simulink model "test"  (R2023b)
settings: Solver=VariableStepAuto  StartTime=0.0  StopTime=10.0  RelTol=1e-3
values from neighbouring files (symbols this model uses):
  f = 50    [model_script.m]    (also in setup_environment.m; test_setup.m)
  l = x./(2*pi*f)    [model_script.m]    (also in setup_environment.m; test_calc.m = 4e-07; test_setup.m = 4e-07)
  l1 = 3    [model_script.m]    (also in setup_environment.m; test_setup.m)
  l2 = 3.5    [model_script.m]    (also in setup_environment.m; test_setup.m = 5)
  l3 = 1.8    [model_script.m]    (also in setup_environment.m; test_setup.m = 8)
  l4 = 15    [test_setup.m]
  L_S = 16E-3    (= 0.016)    [model_script.m]    (also in setup_environment.m; test_setup.m = 0.01658)
  m_actual = 0.2    [model_script.m]    (also in run_sim.m = m_value(jjj); setup_environment.m; test_setup.m = 0.4)
  r = 0.4013    [model_script.m]    (also in setup_environment.m; test_calc.m = 0.4; test_setup.m = 0.4)
  R_S = 0.8913    [model_script.m]    (also in setup_environment.m; test_setup.m = 0.8929)
  trigger = [0 0 0 0]    [test_setup.m]
  V_S = 11000    [model_script.m]    (also in setup_environment.m; test_setup.m)
libraries: spsThreePhaseSeriesRLCBranchLib x8, spsThreePhaseSeriesRLCLoadLib x4, spsThreePhaseFaultLib x4, spsThreePhaseVIMeasurementLib x1, spsThreePhaseSourceLib x1, spsVoltageMeasurementLib x1, sps_lib x1
settings Model: Creator=CoolBose  LastModifiedBy=CoolBose

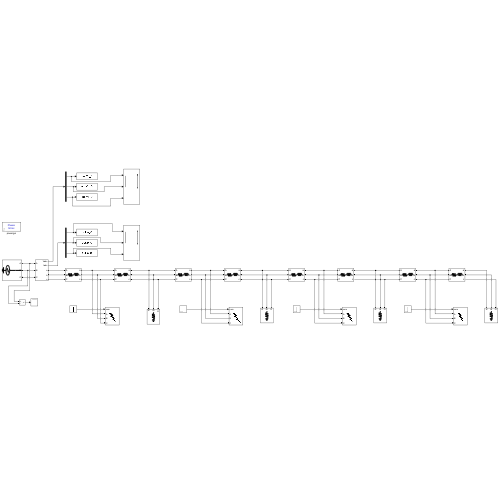
[thumbnail: Simulink's stored preview of the top-level diagram]
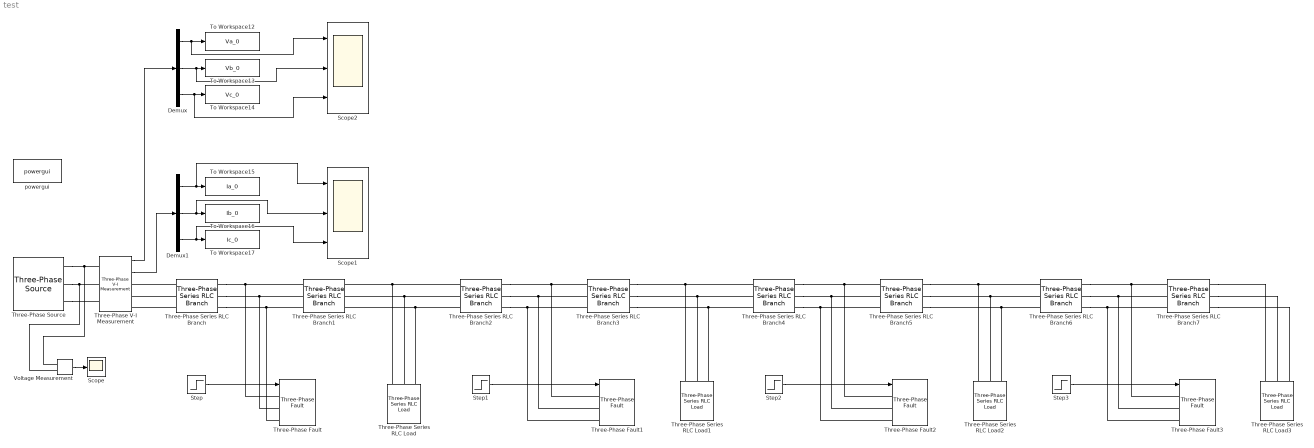
== system test ==
  Demux : Demux  Outputs=3
  Demux1 : Demux  Outputs=3
  Scope : Scope
  Scope1 : Scope  NumInputPorts=3
  Scope2 : Scope  NumInputPorts=3
  Step : Step  Time=5  After=trigger(1)  SampleTime=0
  Step1 : Step  Time=5  After=trigger(2)  SampleTime=0
  Step2 : Step  Time=5  After=trigger(3)  SampleTime=0
  Step3 : Step  Time=5  After=trigger(4)  SampleTime=0
  Three-Phase Series RLC Branch : spsThreePhaseSeriesRLCBranchLib/Three-Phase Series RLC Branch  LConnTagsString=A|B|C  RConnTagsString=A|B|C  BranchType=RL  Resistance=r*l1*m_actual  Inductance=l*l1*m_actual  Capacitance=1e-6  Measurements=None
  Three-Phase Series RLC Branch1 : spsThreePhaseSeriesRLCBranchLib/Three-Phase Series RLC Branch  LConnTagsString=A|B|C  RConnTagsString=A|B|C  BranchType=RL  Resistance=r*l1*(1-m_actual)  Inductance=l*l1*(1-m_actual)  Capacitance=1e-6  Measurements=None
  Three-Phase Series RLC Branch2 : spsThreePhaseSeriesRLCBranchLib/Three-Phase Series RLC Branch  LConnTagsString=A|B|C  RConnTagsString=A|B|C  BranchType=RL  Resistance=r*m_actual*l2  Inductance=l*m_actual*l2  Capacitance=1e-6  Measurements=None
  Three-Phase Series RLC Branch3 : spsThreePhaseSeriesRLCBranchLib/Three-Phase Series RLC Branch  LConnTagsString=A|B|C  RConnTagsString=A|B|C  BranchType=RL  Resistance=r*(1-m_actual)*l2  Inductance=l*(1-m_actual)*l2  Capacitance=1e-6  Measurements=None
  Three-Phase Series RLC Branch4 : spsThreePhaseSeriesRLCBranchLib/Three-Phase Series RLC Branch  LConnTagsString=A|B|C  RConnTagsString=A|B|C  BranchType=RL  Resistance=r*m_actual*l3  Inductance=l*m_actual*l3  Capacitance=1e-6  Measurements=None
  Three-Phase Series RLC Branch5 : spsThreePhaseSeriesRLCBranchLib/Three-Phase Series RLC Branch  LConnTagsString=A|B|C  RConnTagsString=A|B|C  BranchType=RL  Resistance=r*(1-m_actual)*l3  Inductance=l*(1-m_actual)*l3  Capacitance=1e-6  Measurements=None
  Three-Phase Series RLC Branch6 : spsThreePhaseSeriesRLCBranchLib/Three-Phase Series RLC Branch  LConnTagsString=A|B|C  RConnTagsString=A|B|C  BranchType=RL  Resistance=r*m_actual*l4  Inductance=l*m_actual*l4  Capacitance=1e-6  Measurements=None
  Three-Phase Series RLC Branch7 : spsThreePhaseSeriesRLCBranchLib/Three-Phase Series RLC Branch  LConnTagsString=A|B|C  RConnTagsString=A|B|C  BranchType=RL  Resistance=r*(1-m_actual)*l4  Inductance=l*(1-m_actual)*l4  Capacitance=1e-6  Measurements=None
  Three-Phase Series RLC Load : spsThreePhaseSeriesRLCLoadLib/Three-Phase Series RLC Load  LConnTagsString=A|B|C  Configuration=Y (grounded)  NominalVoltage=V_S  Vabc=[1e3 1e3 1e3]  Vabcp=[1e3 1e3 1e3]  NominalFrequency=f  UnbalancedPower=off  ActivePower=P_L1  InductivePower=Q_L1  CapacitivePower=0  Pabc=[10e3 9e3 11e3]  QLabc=[100 90 110]  QCabc=[100 90 110]  Pabcp=[10e3 9e3 11e3]  QLabcp=[100 90 110]  QCabcp=[100 90 110]  Measurements=None  LoadType=constant Z
  Three-Phase Series RLC Load1 : spsThreePhaseSeriesRLCLoadLib/Three-Phase Series RLC Load  LConnTagsString=A|B|C  Configuration=Y (grounded)  NominalVoltage=V_S  Vabc=[1e3 1e3 1e3]  Vabcp=[1e3 1e3 1e3]  NominalFrequency=f  UnbalancedPower=off  ActivePower=P_L2  InductivePower=Q_L2  CapacitivePower=0  Pabc=[10e3 9e3 11e3]  QLabc=[100 90 110]  QCabc=[100 90 110]  Pabcp=[10e3 9e3 11e3]  QLabcp=[100 90 110]  QCabcp=[100 90 110]  Measurements=None  LoadType=constant Z
  Three-Phase Series RLC Load2 : spsThreePhaseSeriesRLCLoadLib/Three-Phase Series RLC Load  LConnTagsString=A|B|C  Configuration=Y (grounded)  NominalVoltage=V_S  Vabc=[1e3 1e3 1e3]  Vabcp=[1e3 1e3 1e3]  NominalFrequency=f  UnbalancedPower=off  ActivePower=P_L3  InductivePower=Q_L3  CapacitivePower=0  Pabc=[10e3 9e3 11e3]  QLabc=[100 90 110]  QCabc=[100 90 110]  Pabcp=[10e3 9e3 11e3]  QLabcp=[100 90 110]  QCabcp=[100 90 110]  Measurements=None  LoadType=constant Z
  Three-Phase Series RLC Load3 : spsThreePhaseSeriesRLCLoadLib/Three-Phase Series RLC Load  LConnTagsString=A|B|C  Configuration=Y (grounded)  NominalVoltage=V_S  Vabc=[1e3 1e3 1e3]  Vabcp=[1e3 1e3 1e3]  NominalFrequency=f  UnbalancedPower=off  ActivePower=P_L4  InductivePower=Q_L4  CapacitivePower=0  Pabc=[10e3 9e3 11e3]  QLabc=[100 90 110]  QCabc=[100 90 110]  Pabcp=[10e3 9e3 11e3]  QLabcp=[100 90 110]  QCabcp=[100 90 110]  Measurements=None  LoadType=constant Z
  Three-Phase V-I Measurement : spsThreePhaseVIMeasurementLib/Three-Phase V-I Measurement  VoltageMeasurement=phase-to-ground  SetLabelV=off  LabelV=Vabc  Vpu=off  VpuLL=off  CurrentMeasurement=yes  SetLabelI=off  LabelI=Iabc  Ipu=off  Pbase=100e6  Vbase=500e3  OutputType=Complex  PhasorSimulation=on  PSBequivalent=0
  Three-Phase Fault : spsThreePhaseFaultLib/Three-Phase Fault  InitialStates=0  FaultA=on  FaultB=off  FaultC=off  GroundFault=on  SwitchTimes="[1/60  5/60]"  External=on  SwitchStatus=NaN  FaultResistance=rf  GroundResistance=0.001  SnubberResistance=1e6  SnubberCapacitance=inf  Measurements=None
  Three-Phase Fault1 : spsThreePhaseFaultLib/Three-Phase Fault  InitialStates=0  FaultA=on  FaultB=on  FaultC=on  GroundFault=on  SwitchTimes="[1/60  5/60]"  External=on  SwitchStatus=NaN  FaultResistance=rf  GroundResistance=0.001  SnubberResistance=1e6  SnubberCapacitance=inf  Measurements=None
  Three-Phase Fault2 : spsThreePhaseFaultLib/Three-Phase Fault  InitialStates=0  FaultA=on  FaultB=on  FaultC=on  GroundFault=on  SwitchTimes="[1/60  5/60]"  External=on  SwitchStatus=NaN  FaultResistance=rf  GroundResistance=0.001  SnubberResistance=1e6  SnubberCapacitance=inf  Measurements=None
  Three-Phase Fault3 : spsThreePhaseFaultLib/Three-Phase Fault  InitialStates=0  FaultA=on  FaultB=on  FaultC=on  GroundFault=on  SwitchTimes="[1/60  5/60]"  External=on  SwitchStatus=NaN  FaultResistance=rf  GroundResistance=0.001  SnubberResistance=1e6  SnubberCapacitance=inf  Measurements=None
  Three-Phase Source : spsThreePhaseSourceLib/Three-Phase Source  InternalConnection=Yg  VoltagePhases=off  Voltage=V_S  PhaseAngle=0  Voltage_phases=[11e3 25e3 25e3]/sqrt(3)  PhaseAngles_phases=[0 -120 +120]  Frequency=f  NonIdealSource=off  SpecifyImpedance=off  Resistance=R_S  Inductance=L_S  ShortCircuitLevel=100e6  BaseVoltage=V_S  XRratio=7  BusType=swing  Pref=10e3  Qref=0  Prefabc=[10e3, 10e3, 10e3]  Qrefabc=[0, 0, 0]  Qmin=-inf  Qmax=inf
  To Workspace12 : ToWorkspace  VariableName=Va_0  SampleTime=-1
  To Workspace13 : ToWorkspace  VariableName=Vb_0  SaveFormat=Structure With Time  SampleTime=-1
  To Workspace14 : ToWorkspace  VariableName=Vc_0  SaveFormat=Structure With Time  SampleTime=-1
  To Workspace15 : ToWorkspace  VariableName=Ia_0  SaveFormat=Structure With Time  SampleTime=-1
  To Workspace16 : ToWorkspace  VariableName=Ib_0  SaveFormat=Structure With Time  SampleTime=-1
  To Workspace17 : ToWorkspace  VariableName=Ic_0  SaveFormat=Structure With Time  SampleTime=-1
  Voltage Measurement : spsVoltageMeasurementLib/Voltage Measurement  PhasorSimulation=on  OutputType=Complex  PSBequivalent=0
  powergui : sps_lib/powergui  Priority=1  SimulationMode=Phasor  SampleTime=50e-6  frequency=50  Iterations=50  frequencyindice=50  Pbase=100e6  ErrMax=1e-4  UnitsV=kV  UnitsW=MW  buscounter=0  FunctionMessages=off  echomessages=off  EnableUseOfTLC=off  CurrentSourceSwitches=off  DisableSnubberDevices=off  DisableRonSwitches=off  DisableVfSwitches=off  DisplayEquations=off  AutomaticDiscreteSolvers=off  SolverType=Tustin/Backward Euler (TBE)  Interpol=off  ExternalGateDelay=off  methode=off  Ts=100  x0status=blocks  SPID=on  SwTol=0  HookPort=off  NonlinearTolerance=1e-4  nMaxIteration=100  ContinueOnMaxIteration=off  RestoreLinks=warning  ResistiveCurrentMeasurement=off  Frange=[0:2:500]  Ylog=off  Xlog=on  ShowGrid=off  save=off  variable=ZData  structure=0  ZoomFFT=off  StartTime=0.0  cycles=1  DisplayStyle=1  fundamental=60  FreqAxis=off  MaxFrequency=1000  frequencyindicesteady=1  RmsSteady=1  display=off
  wires:
  Step/1 -> Three-Phase Fault/1
  Demux/3 -> Scope2/3, To Workspace14/1
  Demux/2 -> Scope2/2, To Workspace13/1
  Demux1/3 -> Scope1/3, To Workspace17/1
  Demux1/1 -> Scope1/1, To Workspace15/1
  Demux/1 -> Scope2/1, To Workspace12/1
  Demux1/2 -> Scope1/2, To Workspace16/1
  Three-Phase V-I Measurement/2 -> Demux1/1
  Three-Phase V-I Measurement/1 -> Demux/1
  Voltage Measurement/1 -> Scope/1
  Step1/1 -> Three-Phase Fault1/1
  Step2/1 -> Three-Phase Fault2/1
  Step3/1 -> Three-Phase Fault3/1
  connections:
  Three-Phase Series RLC Branch/RConn1 -- Three-Phase Fault/LConn1 -- Three-Phase Series RLC Branch1/LConn1
  Three-Phase Series RLC Branch/RConn2 -- Three-Phase Fault/LConn2 -- Three-Phase Series RLC Branch1/LConn2
  Three-Phase Series RLC Branch/RConn3 -- Three-Phase Fault/LConn3 -- Three-Phase Series RLC Branch1/LConn3
  Three-Phase Series RLC Branch2/LConn1 -- Three-Phase Series RLC Branch1/RConn1 -- Three-Phase Series RLC Load/LConn1
  Three-Phase Series RLC Branch2/LConn2 -- Three-Phase Series RLC Branch1/RConn2 -- Three-Phase Series RLC Load/LConn2
  Three-Phase Series RLC Branch2/LConn3 -- Three-Phase Series RLC Branch1/RConn3 -- Three-Phase Series RLC Load/LConn3
  Three-Phase Series RLC Branch/LConn1 -- Three-Phase V-I Measurement/RConn1
  Three-Phase Series RLC Branch/LConn2 -- Three-Phase V-I Measurement/RConn2
  Three-Phase Series RLC Branch/LConn3 -- Three-Phase V-I Measurement/RConn3
  Three-Phase Source/RConn1 -- Voltage Measurement/LConn1 -- Three-Phase V-I Measurement/LConn1
  Three-Phase Source/RConn2 -- Voltage Measurement/LConn2 -- Three-Phase V-I Measurement/LConn2
  Three-Phase Source/RConn3 -- Three-Phase V-I Measurement/LConn3
  Three-Phase Fault1/LConn1 -- Three-Phase Series RLC Branch2/RConn1 -- Three-Phase Series RLC Branch3/LConn1
  Three-Phase Fault1/LConn2 -- Three-Phase Series RLC Branch3/LConn2 -- Three-Phase Series RLC Branch2/RConn2
  Three-Phase Fault1/LConn3 -- Three-Phase Series RLC Branch3/LConn3 -- Three-Phase Series RLC Branch2/RConn3
  Three-Phase Series RLC Branch3/RConn2 -- Three-Phase Series RLC Branch4/LConn2 -- Three-Phase Series RLC Load1/LConn2
  Three-Phase Series RLC Branch3/RConn1 -- Three-Phase Series RLC Branch4/LConn1 -- Three-Phase Series RLC Load1/LConn1
  Three-Phase Series RLC Branch3/RConn3 -- Three-Phase Series RLC Branch4/LConn3 -- Three-Phase Series RLC Load1/LConn3
  Three-Phase Series RLC Branch4/RConn3 -- Three-Phase Fault2/LConn3 -- Three-Phase Series RLC Branch5/LConn3
  Three-Phase Series RLC Branch4/RConn2 -- Three-Phase Fault2/LConn2 -- Three-Phase Series RLC Branch5/LConn2
  Three-Phase Series RLC Branch5/LConn1 -- Three-Phase Fault2/LConn1 -- Three-Phase Series RLC Branch4/RConn1
  Three-Phase Series RLC Branch5/RConn1 -- Three-Phase Series RLC Branch6/LConn1 -- Three-Phase Series RLC Load2/LConn1
  Three-Phase Series RLC Branch5/RConn3 -- Three-Phase Series RLC Branch6/LConn3 -- Three-Phase Series RLC Load2/LConn3
  Three-Phase Series RLC Branch5/RConn2 -- Three-Phase Series RLC Branch6/LConn2 -- Three-Phase Series RLC Load2/LConn2
  Three-Phase Series RLC Branch7/LConn1 -- Three-Phase Fault3/LConn1 -- Three-Phase Series RLC Branch6/RConn1
  Three-Phase Series RLC Branch6/RConn3 -- Three-Phase Fault3/LConn3 -- Three-Phase Series RLC Branch7/LConn3
  Three-Phase Series RLC Branch6/RConn2 -- Three-Phase Fault3/LConn2 -- Three-Phase Series RLC Branch7/LConn2
  Three-Phase Series RLC Branch7/RConn2 -- Three-Phase Series RLC Load3/LConn2
  Three-Phase Series RLC Branch7/RConn1 -- Three-Phase Series RLC Load3/LConn1
  Three-Phase Series RLC Branch7/RConn3 -- Three-Phase Series RLC Load3/LConn3
